simulink model "Linear_MPC_Controller"  (R2024b)
settings: configuration reference "linear_controller_config" (kept outside this file)
libraries: mpclib x1
settings Model: DataDictionary=sim_data_unstable_system.sldd  Creator=tshintai  LastModifiedBy=tshintai
settings ConfigSetRef: SourceName=linear_controller_config

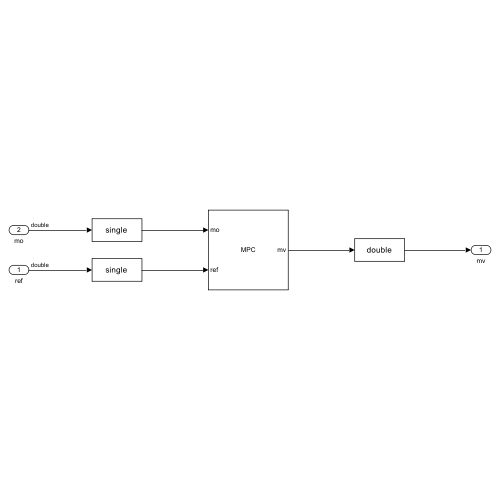
[thumbnail: Simulink's stored preview of the top-level diagram]
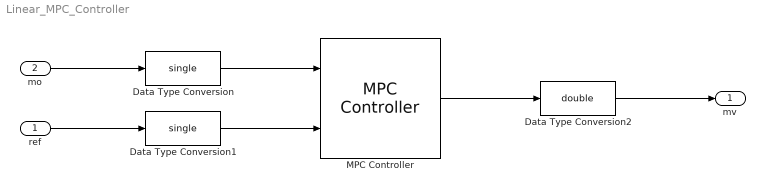
== system Linear_MPC_Controller ==
  ref : Inport  OutDataTypeStr=double
  mo : Inport  Port=2  OutDataTypeStr=double
  Data Type Conversion : DataTypeConversion  OutDataTypeStr=single  SaturateOnIntegerOverflow=off  RndMeth=Floor
  Data Type Conversion1 : DataTypeConversion  OutDataTypeStr=single  SaturateOnIntegerOverflow=off  RndMeth=Floor
  Data Type Conversion2 : DataTypeConversion  OutDataTypeStr=double  SaturateOnIntegerOverflow=off  RndMeth=Floor
  MPC Controller : mpclib/MPC Controller  SCDEnableBlockLinearizationSpecification=on  mpcobj=mpcObj  is_multiple=0  enable_value=0  return_u0=off  updateMPCinCallerWorkspace=on  md_inport=off  mv_inport=off  uref_inport=off  return_cost=off  return_mvseq=off  return_qpstatus=off  return_xseq=off  return_state=off  return_ovseq=off  state_inport=off  umin_inport=off  umax_inport=off  ymin_inport=off  ymax_inport=off  cc_inport=off  ywt_inport=off  uwt_inport=off  duwt_inport=off  rhoeps_inport=off  pm_inport=off  MaximumP=10  HorizonChoice=FixedHorizon  n_ts=0.01  n_p=32  n_mv=1  n_md=0  n_ud=1  n_mo=1  n_uo=0  BlockDataType=single  SampleTimeInherited=off  switch_inport=off
  mv : Outport
  wires:
  ref/1 -> Data Type Conversion1/1
  Data Type Conversion2/1 -> mv/1
  Data Type Conversion/1 -> MPC Controller/1
  mo/1 -> Data Type Conversion/1
  Data Type Conversion1/1 -> MPC Controller/2
  MPC Controller/1 -> Data Type Conversion2/1
